simulink model "mcb_microchip_pmsm_parameter_est_SAME70"  (R2023b)
settings: Solver=FixedStepDiscrete  StartTime=0.0  StopTime=15  RelTol=1e-3  EnableMultiTasking=on
InitFcn:
  | mcb_microchip_pmsm_parameter_est_SAME70_data;
values from neighbouring files (symbols this model uses):
  Ts = T_pwm    (= 5e-05)    [mcb_microchip_pmsm_parameter_est_SAME70_data.m]
  Ts_motor = T_pwm/2    (= 2.5e-05)    [mcb_microchip_pmsm_parameter_est_SAME70_data.m]
undefined symbols (not defined in the file or in its folder): A24, AD10, AD7, ADC0, inverter, LQFP144, MaxPer, ms, ns, PA0, PA1, PA10, PA11, PA12, PA13, PA16, PA18, PA9, PB0, PD18, PD19, PD24, PD25, PD26, PI_params, Pin, pmsm, Resol, SAME70Q21B, target, Unsigned
libraries: simulink x18, MCHP_Blockset x13, mcbpmsmparamestlib x5, svdutilitieslib x4, mcbpositiondecoderlib x3, mcbplantlib x1, autolibpmsmexterior x1, mcbcontrolslib x1
(part 3 of 4)

== system mcb_microchip_pmsm_parameter_est_SAME70/Microcontroller/Heartbeat LED ==
  Codegen : Subsystem  VariantControl=(codegen)
  Sim : Subsystem  VariantControl=(sim)

== system mcb_microchip_pmsm_parameter_est_SAME70/Microcontroller/Input HW Drivers ==
  PhaseCurr_fb : Inport
  Position_fb : Inport  Port=2
  Codegen : Subsystem  VariantControl=(codegen)
  Sim : Subsystem  VariantControl=(sim)
  IabADC : Outport
  VdcADC : Outport  Port=2
  Vabc_ADC : Outport  Port=3
  eQEP : Outport  Port=4

== system mcb_microchip_pmsm_parameter_est_SAME70/Microcontroller/Input Scaling ==
  Mode : Inport
  Iab_ADC : Inport  Port=2
  Vdc_ADC : Inport  Port=3
  Vabc_ADC : Inport  Port=4
  Gain : Gain  Gain=inverter.VoltPerCount  OutDataTypeStr=dataType  RndMeth=Simplest
  Gain1 : Gain  Gain=inverter.VoltPerCount  OutDataTypeStr=dataType  RndMeth=Simplest
  Variant Subsystem : Subsystem  Variant=on
  Iab : Outport
  Vdc : Outport  Port=2
  Vabc : Outport  Port=3
  wires:
  Variant Subsystem/1(Iab) -> Iab/1
  Mode/1 -> Variant Subsystem/1(Mode)
  Iab_ADC/1 -> Variant Subsystem/2(Iab_ADC)
  Vdc_ADC/1 -> Gain/1
  Gain/1 -> Vdc/1
  Vabc_ADC/1 -> Gain1/1
  Gain1/1 -> Vabc/1

== system mcb_microchip_pmsm_parameter_est_SAME70/Microcontroller/Mode Control ==
  ClosedLoop : Subsystem  VariantControl=inverter.ADCOffsetCalibEnable == 0 && pmsm.QEPIndexPresent == true
  CurrentCalib : Subsystem  VariantControl=inverter.ADCOffsetCalibEnable == 1 && pmsm.QEPIndexPresent == true
  CurrentPosCalib : Subsystem  VariantControl=inverter.ADCOffsetCalibEnable == 1 && pmsm.QEPIndexPresent == false
  PosCalib : Subsystem  VariantControl=inverter.ADCOffsetCalibEnable == 0 && pmsm.QEPIndexPresent == false
  Mode : Outport

== system mcb_microchip_pmsm_parameter_est_SAME70/Microcontroller/Output PWM Drivers ==
  PWM_In : Inport
  InvEn : Inport  Port=2
  Codegen : Subsystem  VariantControl=(codegen)
  Sim : Subsystem  VariantControl=(sim)
  PWM : Outport

== system mcb_microchip_pmsm_parameter_est_SAME70/Microcontroller/Output Scaling ==
  Mode : Inport
  Vabc_Ref : Inport  Port=2
  InverterEn : Inport  Port=3
  Constant2 : Constant  OutDataTypeStr=dataType
  Current offset measurement : Constant  Value=[0 0 0]  OutDataTypeStr=dataType
  Mode1 : InportShadow
  Mode2 : InportShadow
  Position offset calibration : Constant  Value=[0.2 -0.1 -0.1]  OutDataTypeStr=dataType
  Switch : Switch  Threshold=1  SaturateOnIntegerOverflow=off  InputSameDT=off
  Switch1 : Switch  Threshold=2  SaturateOnIntegerOverflow=off  InputSameDT=off
  Switch2 : Switch  Threshold=2  SaturateOnIntegerOverflow=off  InputSameDT=off
  PWM : Outport
  InvEn : Outport  Port=2
  wires:
  Switch/1 -> PWM/1
  Switch1/1 -> InvEn/1
  Mode/1 -> Switch/2
  Current offset measurement/1 -> Switch/3
  Switch2/1 -> Switch/1
  Mode1/1 -> Switch2/2
  Vabc_Ref/1 -> Switch2/1
  Position offset calibration/1 -> Switch2/3
  InverterEn/1 -> Switch1/1
  Mode2/1 -> Switch1/2
  Constant2/1 -> Switch1/3

== system mcb_microchip_pmsm_parameter_est_SAME70/Microcontroller/SCI In Abstraction ==
  SCI_Data : Inport
  Mode : Inport  Port=2
  Variant Subsystem : Subsystem  Variant=on  VariantControlMode=sim codegen switching
  ConfigAndCommand : Outport
  DebugSel : Outport  Port=2
  wires:
  Variant Subsystem/1(ConfigAndCommand) -> ConfigAndCommand/1
  Variant Subsystem/2(DebugSel) -> DebugSel/1
  SCI_Data/1 -> Variant Subsystem/1(SCI_Data)
  Mode/1 -> Variant Subsystem/2(Mode)

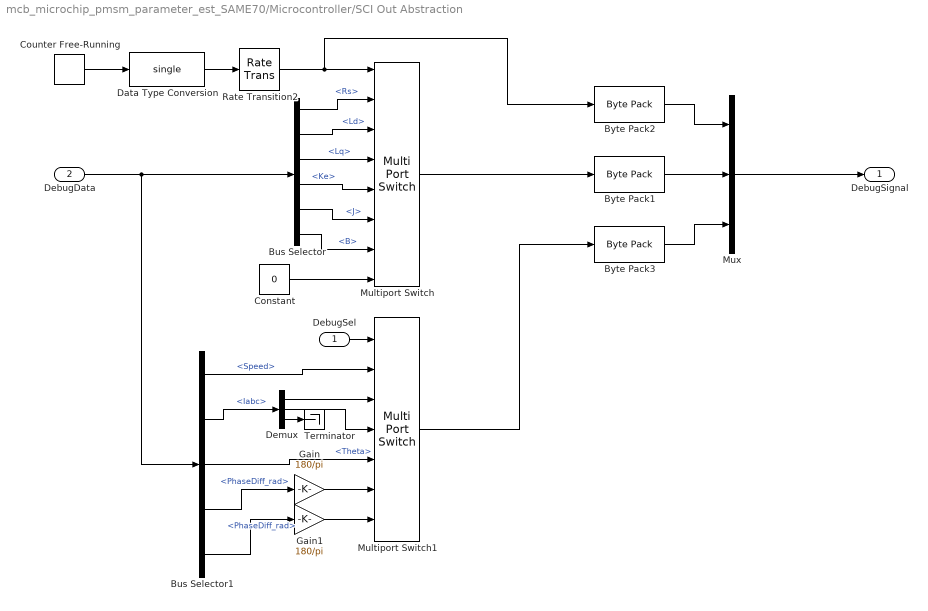
== system mcb_microchip_pmsm_parameter_est_SAME70/Microcontroller/SCI Out Abstraction ==
  DebugSel : Inport
  DebugData : Inport  Port=2
  Bus Selector : BusSelector  OutputSignals=MotorParams.Rs,MotorParams.Ld,MotorParams.Lq,MotorParams.Ke,MotorParams.J,MotorParams.B
  Bus Selector1 : BusSelector  OutputSignals=HWInputs.Speed,HWInputs.Iabc,HWInputs.Theta,LdLog.PhaseDiff_rad,LqLog.PhaseDiff_rad
  Byte Pack1 : svdutilitieslib/Byte Pack  maskPackedDataType=uint8  datatypes={'single'}  byteAlign=1  blockPlatform=tic2000
  Byte Pack2 : svdutilitieslib/Byte Pack  maskPackedDataType=uint8  datatypes={'single'}  byteAlign=1  blockPlatform=tic2000
  Byte Pack3 : svdutilitieslib/Byte Pack  maskPackedDataType=uint8  datatypes={'single'}  byteAlign=1  blockPlatform=tic2000
  Constant : Constant  Value=0  OutDataTypeStr=dataType
  Counter Free-Running : simulink/Sources/Counter Free-Running  NumBits=3  tsamp=0.5
  Data Type Conversion : DataTypeConversion  OutDataTypeStr=single  RndMeth=Simplest  SaturateOnIntegerOverflow=off
  Demux : Demux  Outputs=3
  Gain : Gain  Gain=180/pi
  Gain1 : Gain  Gain=180/pi
  Multiport Switch : MultiPortSwitch  Inputs=7  DiagnosticForDefault=None  SaturateOnIntegerOverflow=off  InputSameDT=off
  Multiport Switch1 : MultiPortSwitch  Inputs=6  DiagnosticForDefault=None  SaturateOnIntegerOverflow=off  InputSameDT=off
  Mux : Mux  Inputs=3
  Rate Transition2 : RateTransition  Deterministic=off  OutPortSampleTime=Ts
  Terminator : Terminator
  DebugSignal : Outport
  wires:
  Counter Free-Running/1 -> Data Type Conversion/1
  Data Type Conversion/1 -> Rate Transition2/1
  DebugData/1 -> Bus Selector1/1, Bus Selector/1
  Bus Selector/4 -> Multiport Switch/5  "<Ke>"
  Bus Selector/5 -> Multiport Switch/6  "<J>"
  Bus Selector/3 -> Multiport Switch/4  "<Lq>"
  Bus Selector/6 -> Multiport Switch/7  "<B>"
  Bus Selector/2 -> Multiport Switch/3  "<Ld>"
  Bus Selector/1 -> Multiport Switch/2  "<Rs>"
  Constant/1 -> Multiport Switch/8
  DebugSel/1 -> Multiport Switch1/1
  Multiport Switch/1 -> Byte Pack1/1
  Multiport Switch1/1 -> Byte Pack3/1
  Bus Selector1/1 -> Multiport Switch1/2  "<Speed>"
  Demux/1 -> Multiport Switch1/3
  Demux/2 -> Multiport Switch1/4
  Mux/1 -> DebugSignal/1
  Demux/3 -> Terminator/1
  Byte Pack2/1 -> Mux/1
  Byte Pack1/1 -> Mux/2
  Byte Pack3/1 -> Mux/3
  Rate Transition2/1 -> Byte Pack2/1, Multiport Switch/1
  Gain/1 -> Multiport Switch1/6
  Gain1/1 -> Multiport Switch1/7
  Bus Selector1/4 -> Gain/1  "<PhaseDiff_rad>"
  Bus Selector1/5 -> Gain1/1  "<PhaseDiff_rad>"
  Bus Selector1/2 -> Demux/1  "<Iabc>"
  Bus Selector1/3 -> Multiport Switch1/5  "<Theta>"

== system mcb_microchip_pmsm_parameter_est_SAME70/Microcontroller/SCI_Rx ==
  CodeGen : Subsystem
  Sim : Subsystem
  Variant Source : VariantSource  VariantControlMode=sim codegen switching
  Data : Outport
  wires:
  CodeGen/1(Data) -> Variant Source/1
  Variant Source/1 -> Data/1
  Sim/1(Data) -> Variant Source/2

== system mcb_microchip_pmsm_parameter_est_SAME70/Microcontroller/SCI_Tx ==
  SCI_Tx_Data : Inport
  Codegen : Subsystem  SystemSampleTime=0.03  VariantControl=(codegen)
  Sim : Subsystem  VariantControl=(sim)

== system mcb_microchip_pmsm_parameter_est_SAME70/Inverter and Motor/Inverter and Motor/Codegen ==
  Duty_Cycles : Inport
  Ground : Ground
  Terminator : Terminator
  PhaseCurr_fb : Outport
  Position_fb : Outport  Port=2
  wires:
  Duty_Cycles/1 -> Terminator/1
  Ground/1 -> PhaseCurr_fb/1, Position_fb/1

== system mcb_microchip_pmsm_parameter_est_SAME70/Inverter and Motor/Inverter and Motor/Sim ==
  Duty_Cycles : Inport
  Motor : Subsystem
  RT1 : RateTransition  Deterministic=off  OutPortSampleTime=Ts_simulink
  RT2 : RateTransition  Deterministic=off  OutPortSampleTime=Ts_simulink
  Rate Transition2 : RateTransition  Deterministic=off  OutPortSampleTime=Ts
  Rate Transition3 : RateTransition  Deterministic=off  OutPortSampleTime=Ts_inverter
  Rate Transition4 : RateTransition  Deterministic=off  OutPortSampleTime=Ts
  Sensor Measurements : Subsystem
  PhaseCurr_fb : Outport
  Position_fb : Outport  Port=2
  wires:
  RT1/1 -> Sensor Measurements/2(PhaseCurr)
  Duty_Cycles/1 -> Rate Transition3/1
  Sensor Measurements/2(Position_fb) -> Rate Transition4/1
  Sensor Measurements/1(PhaseCurr_fb) -> Rate Transition2/1
  Rate Transition2/1 -> PhaseCurr_fb/1
  Rate Transition4/1 -> Position_fb/1
  RT2/1 -> Sensor Measurements/1(Info)
  Rate Transition3/1 -> Motor/1(Duty_Cycles)
  Motor/1(ThetaMech) -> RT2/1
  Motor/2(Iabc) -> RT1/1

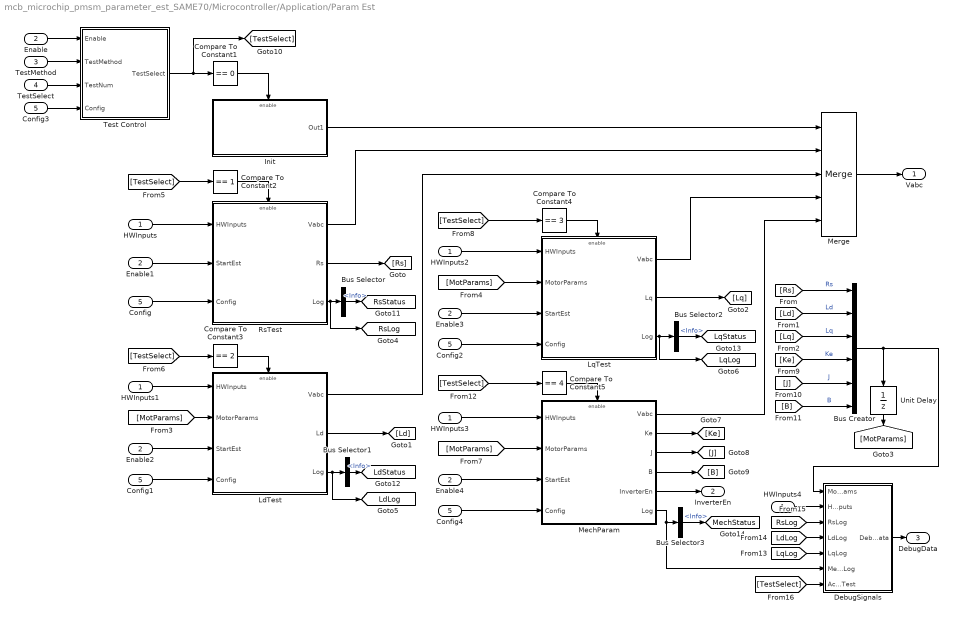
== system mcb_microchip_pmsm_parameter_est_SAME70/Microcontroller/Application/Param Est ==
  HWInputs : Inport
  Enable : Inport  Port=2
  TestMethod : Inport  Port=3
  TestSelect : Inport  Port=4
  Config : Inport  Port=5
  Bus Creator : BusCreator  Inputs=6
  Bus Selector{,1..3} (4 alike) : BusSelector  OutputSignals=Info
  Compare To Constant1 : simulink/Logic and Bit Operations/Compare To Constant  relop===  const=0  OutDataTypeStr=boolean
  Compare To Constant2 : simulink/Logic and Bit Operations/Compare To Constant  relop===  const=1  OutDataTypeStr=boolean
  Compare To Constant3 : simulink/Logic and Bit Operations/Compare To Constant  relop===  const=2  OutDataTypeStr=boolean
  Compare To Constant4 : simulink/Logic and Bit Operations/Compare To Constant  relop===  const=3  OutDataTypeStr=boolean
  Compare To Constant5 : simulink/Logic and Bit Operations/Compare To Constant  relop===  const=4  OutDataTypeStr=boolean
  Config{1..4} (4 alike) : InportShadow  Port=5
  DebugSignals : Subsystem
  Enable{1..4} (4 alike) : InportShadow  Port=2
  HWInputs{1..4} (4 alike) : InportShadow
  Init : Subsystem
  LdTest : Subsystem
  LqTest : Subsystem
  MechParam : Subsystem
  Merge : Merge  Inputs=5
  RsTest : Subsystem
  Test Control : Subsystem
  Unit Delay : UnitDelay  SampleTime=-1  HasFrameUpgradeWarning=on
  Vabc : Outport
  InverterEn : Outport  Port=2
  DebugData : Outport  Port=3
  tag scope: LdLog=global, LdStatus=global, LqLog=global, LqStatus=global, MechStatus=global, RsLog=global, RsStatus=global
  wires:
  Config/1 -> RsTest/3(Config)
  Config1/1 -> LdTest/4(Config)
  Config2/1 -> LqTest/4(Config)
  HWInputs/1 -> RsTest/1(HWInputs)
  HWInputs1/1 -> LdTest/1(HWInputs)
  HWInputs2/1 -> LqTest/1(HWInputs)
  Bus Creator/1 -> Unit Delay/1, DebugSignals/1(MotorParams)
  RsTest/2(Rs) -> [Rs]
  LdTest/3(Log) -> [LdLog], Bus Selector1/1
  LdTest/2(Ld) -> [Ld]
  LqTest/2(Lq) -> [Lq]
  LqTest/3(Log) -> [LqLog], Bus Selector2/1
  [Rs] -> Bus Creator/1  "Rs"
  [Ld] -> Bus Creator/2  "Ld"
  [Lq] -> Bus Creator/3  "Lq"
  Unit Delay/1 -> [MotParams]
  [MotParams] -> LdTest/2(MotorParams)
  [MotParams] -> LqTest/2(MotorParams)
  Test Control/1(TestSelect) -> [TestSelect], Compare To Constant1/1
  Compare To Constant1/1 -> Init/Enable
  Compare To Constant2/1 -> RsTest/Enable
  Compare To Constant3/1 -> LdTest/Enable
  Compare To Constant4/1 -> LqTest/Enable
  Bus Selector1/1 -> [LdStatus]  "<Info>"
  Bus Selector2/1 -> [LqStatus]  "<Info>"
  Compare To Constant5/1 -> MechParam/Enable
  HWInputs3/1 -> MechParam/1(HWInputs)
  Config4/1 -> MechParam/4(Config)
  [MotParams] -> MechParam/2(MotorParams)
  MechParam/6(Log) -> DebugSignals/6(MechLog), Bus Selector3/1
  MechParam/2(Ke) -> [Ke]
  [Ke] -> Bus Creator/4  "Ke"
  Merge/1 -> Vabc/1
  Init/1(Out1) -> Merge/1
  RsTest/1(Vabc) -> Merge/2
  LdTest/1(Vabc) -> Merge/3
  LqTest/1(Vabc) -> Merge/4
  MechParam/1(Vabc) -> Merge/5
  MechParam/3(J) -> [J]
  MechParam/4(B) -> [B]
  [J] -> Bus Creator/5  "J"
  [B] -> Bus Creator/6  "B"
  MechParam/5(InverterEn) -> InverterEn/1
  Enable/1 -> Test Control/1(Enable)
  TestSelect/1 -> Test Control/3(TestNum)
  TestMethod/1 -> Test Control/2(TestMethod)
  [TestSelect] -> Compare To Constant2/1
  [TestSelect] -> Compare To Constant3/1
  [TestSelect] -> Compare To Constant4/1
  [TestSelect] -> Compare To Constant5/1
  Enable1/1 -> RsTest/2(StartEst)
  Enable2/1 -> LdTest/3(StartEst)
  Enable3/1 -> LqTest/3(StartEst)
  Enable4/1 -> MechParam/3(StartEst)
  Bus Selector/1 -> [RsStatus]  "<Info>"
  Bus Selector3/1 -> [MechStatus]  "<Info>"
  HWInputs4/1 -> DebugSignals/2(HWInputs)
  RsTest/3(Log) -> [RsLog], Bus Selector/1
  [LqLog] -> DebugSignals/5(LqLog)
  [LdLog] -> DebugSignals/4(LdLog)
  [RsLog] -> DebugSignals/3(RsLog)
  DebugSignals/1(DebugData) -> DebugData/1
  Config3/1 -> Test Control/4(Config)
  [TestSelect] -> DebugSignals/7(ActiveTest)

== system mcb_microchip_pmsm_parameter_est_SAME70/Microcontroller/Application Abstraction/Variant Subsystem ==
  eQEPCnt : Inport
  eQEPIndex : Inport  Port=2
  Mode : Inport  Port=3
  Index Absent : Subsystem  VariantControl=pmsm.QEPIndexPresent == false
  Index Present : Subsystem  VariantControl=pmsm.QEPIndexPresent == true
  Theta : Outport
  Speed : Outport  Port=2
  EnClosedLoop : Outport  Port=3

== system mcb_microchip_pmsm_parameter_est_SAME70/Microcontroller/Heartbeat LED/Codegen ==
  DBG LED 1 : MCHP_Blockset/Digital IO/Digital Output Write  PORT=Dynamic Options  PORT_TXT="C   [ 0 : 31 ]"  PIN=23  PACK=off  SIMULTANEOUS=off  ORDERING=None  SampleTime=-1  MCHP_PORT={Digital Out}{DOU}1:1:C23;  MCHP_MASTERLINK=mcb_microchip_pmsm_parameter_est_SAME70_23b_lib/Microcontroller/Configurations/Microchip Master
      settings: SourceProductName=MPLAB Device Blocks for Simulink
  Delay 10Hz : Delay  DelayLength=1  InitialCondition=0  SampleTime=0.25
  Logical Operator : Logic  Operator=NOT  AllPortsSameDT=off  OutDataTypeStr=boolean
  wires:
  Delay 10Hz/1 -> Logical Operator/1
  Logical Operator/1 -> DBG LED 1/1, Delay 10Hz/1

== system mcb_microchip_pmsm_parameter_est_SAME70/Microcontroller/Heartbeat LED/Sim ==

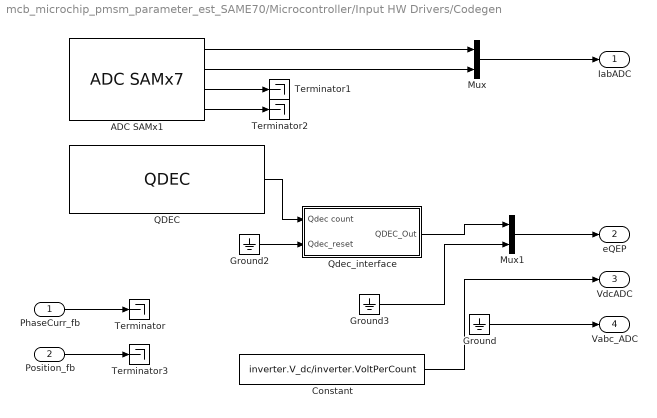
== system mcb_microchip_pmsm_parameter_est_SAME70/Microcontroller/Input HW Drivers/Codegen ==
  PhaseCurr_fb : Inport
  Position_fb : Inport  Port=2
  ADC SAMx1 : MCHP_Blockset/Analog IO/ADC SAMx7  Priority=-2000  AFECx=AFE Controller 0  SIGNMODE_SingleEnded=Unsigned (uint16)  SIGNMODE_Differential=Unsigned (uint16)  AFEC0_seq0=Dynamic Options  AFEC0_seq0_TXT="AD0 / PD30   &   AD6 / PA17"  AFEC1_seq0=Dynamic Options  AFEC1_seq0_TXT=Not used  AFEC0_seq1=Dynamic Options  AFEC0_seq1_TXT=AD7 / PA18  AFEC1_seq1=Dynamic Options  AFEC1_seq1_TXT=Not used  AFEC0_seq2=Dynamic Options  AFEC0_seq2_TXT=AD10 / PB0  AFEC1_seq2=Dynamic Options  AFEC1_seq2_TXT=Not used  AFEC0_seq3=Dynamic Options  AFEC0_seq3_TXT=Not used  AFEC1_seq3=Dynamic Options  AFEC1_seq3_TXT=Not used  AFEC0_seq4=Dynamic Options  AFEC0_seq4_TXT=Not used  AFEC1_seq4=Dynamic Options  AFEC1_seq4_TXT=Not used  AFEC0_seq5=Dynamic Options  AFEC0_seq5_TXT=Not used  AFEC1_seq5=Dynamic Options  AFEC1_seq5_TXT=Not used  AFEC0_seq6=Dynamic Options  AFEC0_seq6_TXT=Not used  AFEC1_seq6=Dynamic Options  AFEC1_seq6_TXT=Not used  AFEC0_seq7=Dynamic Options  AFEC0_seq7_TXT=Not used  AFEC1_seq7=Dynamic Options  AFEC1_seq7_TXT=Not used  AFEC0_seq8=Dynamic Options  AFEC0_seq8_TXT=Not used  AFEC1_seq8=Dynamic Options  AFEC1_seq8_TXT=Not used  AFEC0_seq9=Dynamic Options  AFEC0_seq9_TXT=Not used  AFEC1_seq9=Dynamic Options  AFEC1_seq9_TXT=Not used  AFEC0_seq10=Dynamic Options  AFEC0_seq10_TXT=Not used  AFEC1_seq10=Dynamic Options  AFEC1_seq10_TXT=Not used  AFEC0_seq11=Dynamic Options  AFEC0_seq11_TXT=Not used  AFEC1_seq11=Dynamic Options  AFEC1_seq11_TXT=Not used  SampleTime=Ts  S_INPUT=[-1]  S_INPUT_Size=[3]  S_OUTPUT=[]  S_OUTPUT_Size=[]  S_ListCustomDatatype=S.S_ListCustomDatatype={};  MCHP_AFECC_CLOCK_REQUEST=''  MCHP_AFECC_CLOCK_RESULT=''  MCHP_USER_INTERRUPTS=0  MCHP_PORT={AD0 AFEC0}{AD0}15:2:P126;{AD6 AFEC0}{AD6}15:2:P17;{AD7 AFEC0}{AD7}15:2:P18;{AD10 AFEC0}{AD10}15:2:P32;  MCHP_MASTERLINK=mcb_microchip_pmsm_parameter_est_SAME70_23b_lib/Microcontroller/Configurations/Microchip Master  Rin=< 200 Ohm  RES=12-bit Standard  AFEC0_Synchronisation=Triggered by user defined source  AFEC0_Trig=PWM0 event line 0  AFEC0_TrigTimeStep=on  AFEC1_Synchronisation=Triggered by user defined source  AFEC1_Trig=PWM1 event line 0  AFEC1_TrigTimeStep=off  ADC_TrigInfo=0  AFEC0_seq0_GAIN=1  AFEC1_seq0_GAIN=1  AFEC0_seq1_GAIN=1  AFEC1_seq1_GAIN=1  AFEC0_seq2_GAIN=1  AFEC1_seq2_GAIN=1  AFEC0_seq3_GAIN=1  AFEC1_seq3_GAIN=1  AFEC0_seq4_GAIN=1  AFEC1_seq4_GAIN=1  AFEC0_seq5_GAIN=1  AFEC1_seq5_GAIN=1  AFEC0_seq6_GAIN=1  AFEC1_seq6_GAIN=1  AFEC0_seq7_GAIN=1  AFEC1_seq7_GAIN=1  AFEC0_seq8_GAIN=1  AFEC1_seq8_GAIN=1  AFEC0_seq9_GAIN=1  AFEC1_seq9_GAIN=1  AFEC0_seq10_GAIN=1  AFEC1_seq10_GAIN=1  AFEC0_seq11_GAIN=1  AFEC1_seq11_GAIN=1  AFEC0_seq0_OFFSET=0  AFEC1_seq0_OFFSET=0  AFEC0_seq1_OFFSET=0  AFEC1_seq1_OFFSET=0  AFEC0_seq2_OFFSET=0  AFEC1_seq2_OFFSET=0  AFEC0_seq3_OFFSET=0  AFEC1_seq3_OFFSET=0  AFEC0_seq4_OFFSET=0  AFEC1_seq4_OFFSET=0  AFEC0_seq5_OFFSET=0  AFEC1_seq5_OFFSET=0  AFEC0_seq6_OFFSET=0  AFEC1_seq6_OFFSET=0  AFEC0_seq7_OFFSET=0  AFEC1_seq7_OFFSET=0  AFEC0_seq8_OFFSET=0  AFEC1_seq8_OFFSET=0  AFEC0_seq9_OFFSET=0  AFEC1_seq9_OFFSET=0  AFEC0_seq10_OFFSET=0  AFEC1_seq10_OFFSET=0  AFEC0_seq11_OFFSET=0  AFEC1_seq11_OFFSET=0
      settings: SourceProductName=MPLAB Device Blocks for Simulink
  Constant : Constant  Value=inverter.V_dc/inverter.VoltPerCount  OutDataTypeStr=uint16
  Ground : Ground
  Ground2 : Ground
  Ground3 : Ground
  Mux : Mux  Inputs=2
  Mux1 : Mux  Inputs=2
  QDEC : MCHP_Blockset/QEI/QDEC  QDEC_REF=Dynamic Options  QDEC_REF_TXT=TC0  PHA_PIN=Dynamic Options  PHA_PIN_TXT=PA0 / Pin[102]  PHB_PIN=Dynamic Options  PHB_PIN_TXT=PA1 / Pin[99]  IDX_PIN=Dynamic Options  IDX_PIN_TXT=PA16 / Pin[45]  INVERT_PHA=off  INVERT_PHB=off  INVERT_IDX=off  SWAP_PHA_PHB=off  SampleTime=Ts  MCHP_PORT={TC0}{TIOA0}3:0:P0;{TC0}{TIOB0}3:0:P1;{TC0}{TIOB1}3:0:P16;  MCHP_MASTERLINK=mcb_microchip_pmsm_parameter_est_SAME70_23b_lib/Microcontroller/Configurations/Microchip Master  MCHP_TIMER_REQUEST={Quadrature Decoder (Phase Counter)}{QDEC0}20:4:4:0:[1]:65535;{Quadrature Decoder (IDX Counter)}{QDEC0}20:4:4:0:[2]:65535;{Quadrature Decoder (Speed Measurement Time Base)}{QDEC0}20:4:4:0:[3]:65535;  MCHP_TIMER_RESULT=[1 65535]  QDEC_MODE=Position  POSITION_OUTPUT=is a 16 bits unsigned block output  INDEX_OUTPUT=is not a block output  RESET_INPUT=off  POSITION_RESET_MODE=never reset position  RESET_EDGE=rising edge  POSITION_RESET_VALUE=65535  SPEED_TIME_BASE=Dynamic Options  SPEED_TIME_BASE_TXT=Resol: 53.33(ns) - MaxPer: 3.5(ms)  SPEED_OUTPUT=is a 16 bits unsigned block output  DIR_OUTPUT=is not a block output  DIRCHG_OUTPUT=is not a block output  AUTO_CORRECTION=off  MAX_PERIOD_FILTER=Dynamic Options  MAX_PERIOD_FILTER_TXT=420(ns)  MAXCMP=disabled  MPE_OUTPUT=is not a block output  QERR_OUTPUT=is not a block output
      settings: SourceProductName=MPLAB Device Blocks for Simulink
  Qdec_interface : Subsystem  mask{EnCountPerRev=pmsm.QEPSlits*4}
      mask prompts: EnCountPerRev "Encoder counts per rev"
  Terminator{,1..3} (4 alike) : Terminator
  IabADC : Outport
  eQEP : Outport  Port=2
  VdcADC : Outport  Port=3
  Vabc_ADC : Outport  Port=4
  wires:
  ADC SAMx1/4 -> Terminator2/1
  ADC SAMx1/3 -> Terminator1/1
  Ground2/1 -> Qdec_interface/2(Qdec_reset)
  QDEC/1 -> Qdec_interface/1(Qdec count)
  PhaseCurr_fb/1 -> Terminator/1
  Position_fb/1 -> Terminator3/1
  Ground/1 -> Vabc_ADC/1
  Constant/1 -> VdcADC/1
  ADC SAMx1/1 -> Mux/1
  ADC SAMx1/2 -> Mux/2
  Mux/1 -> IabADC/1
  Qdec_interface/1(QDEC_Out) -> Mux1/1
  Mux1/1 -> eQEP/1
  Ground3/1 -> Mux1/2

== system mcb_microchip_pmsm_parameter_est_SAME70/Microcontroller/Input HW Drivers/Sim ==
  PhaseCurr_fb : Inport
  Position_fb : Inport  Port=2
  Constant : Constant  Value=inverter.V_dc/inverter.VoltPerCount  OutDataTypeStr=uint16
  Ground : Ground
  IabADC : Outport
  eQEP : Outport  Port=2
  VdcADC : Outport  Port=3
  Vabc_ADC : Outport  Port=4
  wires:
  PhaseCurr_fb/1 -> IabADC/1
  Position_fb/1 -> eQEP/1
  Ground/1 -> Vabc_ADC/1
  Constant/1 -> VdcADC/1

== system mcb_microchip_pmsm_parameter_est_SAME70/Microcontroller/Input Scaling/Variant Subsystem ==
  Mode : Inport
  Iab_ADC : Inport  Port=2
  Automatic offset calibration : Subsystem  VariantControl=inverter.ADCOffsetCalibEnable == 1
  Offser via parameter : Subsystem  VariantControl=inverter.ADCOffsetCalibEnable == 0
  Iab : Outport

== system mcb_microchip_pmsm_parameter_est_SAME70/Microcontroller/Mode Control/ClosedLoop ==
  Constant : Constant  Value=2  OutDataTypeStr=single  SampleTime=0.1
  Mode : Outport
  wires:
  Constant/1 -> Mode/1

== system mcb_microchip_pmsm_parameter_est_SAME70/Microcontroller/Mode Control/CurrentCalib ==
  Step : Step  After=2  OutDataTypeStr=single  SampleTime=0.1
  Mode : Outport
  wires:
  Step/1 -> Mode/1

== system mcb_microchip_pmsm_parameter_est_SAME70/Microcontroller/Mode Control/CurrentPosCalib ==
  Add : Sum
  Step : Step  OutDataTypeStr=single  SampleTime=0.1
  Step1 : Step  Time=2  OutDataTypeStr=single  SampleTime=0.1
  Mode : Outport
  wires:
  Step/1 -> Add/1
  Step1/1 -> Add/2
  Add/1 -> Mode/1

== system mcb_microchip_pmsm_parameter_est_SAME70/Microcontroller/Mode Control/PosCalib ==
  Step : Step  Before=1  After=2  OutDataTypeStr=single  SampleTime=0.1
  Mode : Outport
  wires:
  Step/1 -> Mode/1

== system mcb_microchip_pmsm_parameter_est_SAME70/Microcontroller/Output PWM Drivers/Codegen ==
  PWM_In : Inport
  InvEn : Inport  Port=2
  Constant : Constant  Value=0xF000F  OutDataTypeStr=uint32  SampleTime=-1
  Constant1 : Constant  Value=0  OutDataTypeStr=uint32  SampleTime=-1
  Constant2 : Constant  Value=0  OutDataTypeStr=uint32  SampleTime=-1
  Data Type Conversion : DataTypeConversion  OutDataTypeStr=single  SaturateOnIntegerOverflow=off  RndMeth=Floor
  Ground : Ground
  InvEn1 : InportShadow  Port=2
  Mux3 : Mux  Inputs=3
  PWM SAM7x : MCHP_Blockset/PWM IO/PWM SAM7x  Priority=-2000  PWMx=PWM Controller 0  MaxPeriod_s=Ts  PWM0_pinH0=Dynamic Options  PWM0_pinH0_TXT=PA11 / Pin[64]  PWM0_pinL0=Dynamic Options  PWM0_pinL0_TXT=PD24 / Pin[55]  PWM0_pinH1=Dynamic Options  PWM0_pinH1_TXT=PA12 / Pin[68]  PWM0_pinL1=Dynamic Options  PWM0_pinL1_TXT=PD25 / Pin[52]  PWM0_pinH2=Dynamic Options  PWM0_pinH2_TXT=PA13 / Pin[42]  PWM0_pinL2=Dynamic Options  PWM0_pinL2_TXT=PD26 / Pin[53]  PWM0_pinH3=Dynamic Options  PWM0_pinH3_TXT=Not Used  PWM0_pinL3=Dynamic Options  PWM0_pinL3_TXT=Not Used  PWM1_pinH0=Dynamic Options  PWM1_pinH0_TXT=Not Used  PWM1_pinL0=Dynamic Options  PWM1_pinL0_TXT=Not Used  PWM1_pinH1=Dynamic Options  PWM1_pinH1_TXT=Not Used  PWM1_pinL1=Dynamic Options  PWM1_pinL1_TXT=Not Used  PWM1_pinH2=Dynamic Options  PWM1_pinH2_TXT=Not Used  PWM1_pinL2=Dynamic Options  PWM1_pinL2_TXT=Not Used  PWM1_pinH3=Dynamic Options  PWM1_pinH3_TXT=Not Used  PWM1_pinL3=Dynamic Options  PWM1_pinL3_TXT=Not Used  PWM_Centered=on  PWM_SyncWithPWM0=on  PushPull_Mode=off  SampleTime=Ts  S_INPUT=[-1]  S_INPUT_Size=[3]  S_OUTPUT=[]  S_OUTPUT_Size=[]  S_ListCustomDatatype=S.S_ListCustomDatatype={};  evalin_ws=PWM0max0=MCHP_Fun.Hex2num('40AD4C0000000000');PWM1max0=MCHP_Fun.Hex2num('40AD4C0000000000');PWM2max0=MCHP_Fun.Hex2num('40AD4C0000000000');  MCHP_PWMC_CLOCK_REQUEST=''  MCHP_PWMC_CLOCK_RESULT=''  MCHP_USER_INTERRUPTS=0  MCHP_PORT={PWM0H0 }{PWMH0}4:1:P11;{PWM0L0 }{PWML0}4:1:P120;{PWM0H1 }{PWMH1}4:1:P12;{PWM0L1 }{PWML1}4:1:P121;{PWM0H2 }{PWMH2}4:1:P13;{PWM0L2 }{PWML2}4:1:P122;  MCHP_MASTERLINK=mcb_microchip_pmsm_parameter_est_SAME70_23b_lib/Microcontroller/Configurations/Microchip Master  invert_PWMH0=off  invert_PWML0=off  invert_PWMH1=off  invert_PWML1=off  invert_PWMH2=off  invert_PWML2=off  invert_PWMH3=off  invert_PWML3=off  InitPeriod_s=Ts  InitDutyCycle_s=0  InitDeadTimeH_s=1e-6  InitDeadTimeL_s=1e-6  InitEventLine0_ComparatorValue_s=1e-7  InitEventLine1_ComparatorValue_s=[]  BlockInput_VectorScalar=Vectors (grouped by function)  BlockInput_Period=Not a block input  BlockInput_DutyCycle=a Floating Point input within range [-1 1]  BlockInput_DeadTime=Not a block input  BlockInput_OutputOverride=Not a block input  Fault_FPV0=Not forced  Fault_FPV1=Not forced  Fault_FPV2=Not forced  Fault_FPV3=Not forced  Fault_Input0=does nothing  Fault_Input0_FFIL=off  Fault_Input1=does nothing  Fault_Input1_FFIL=off  Fault_Input2=does nothing  Fault_Input2_FFIL=on  Fault_Input3=does nothing  Fault_Input3_FFIL=off  Fault_Input4=does nothing  Fault_Input4_FFIL=on  Fault_Input5=does nothing  Fault_Input5_FFIL=on  Fault_Input6=does nothing  Fault_Input6_FFIL=on  Fault_Input7=does nothing  Fault_Input7_FFIL=on
      settings: SourceProductName=MPLAB Device Blocks for Simulink
  PWM SAM7x Output Override : MCHP_Blockset/PWM IO/PWM SAM7x  Output Override  Priority=-2000  PWMx=PWM Controller 0  SampleTime=Ts  S_INPUT=[-1]  S_INPUT_Size=[3]  S_OUTPUT=[]  S_OUTPUT_Size=[]  S_ListCustomDatatype=S.S_ListCustomDatatype={};  MCHP_MASTERLINK=mcb_microchip_pmsm_parameter_est_SAME70_23b_lib/Microcontroller/Configurations/Microchip Master  Init_PWM_OS=0x0000  Init_PWM_OOV=0x0000  Input_PWM_OS=on  Input_PWM_OS_off=off  Input_PWM_OSS=off  Input_PWM_OSS_off=off  Input_PWM_OSSUPD=off  Input_PWM_OSSUPD_off=off  Input_PWM_OSC=off  Input_PWM_OSC_off=off  Input_PWM_OSCUPD=off  Input_PWM_OSCUPD_off=off  Input_PWM_OOV=on
      settings: SourceProductName=MPLAB Device Blocks for Simulink
  Switch1 : Switch  Threshold=0.5  RndMeth=Simplest  SaturateOnIntegerOverflow=off  InputSameDT=off
  Switch4 : Switch  Threshold=0.5  RndMeth=Simplest  SaturateOnIntegerOverflow=off  InputSameDT=off
  stop : Constant  Value=0  OutDataTypeStr=dataType
  PWM : Outport
  wires:
  Mux3/1 -> Switch4/3
  Switch4/1 -> Data Type Conversion/1
  Data Type Conversion/1 -> PWM SAM7x/1
  stop/1 -> Mux3/3, Mux3/2, Mux3/1
  Ground/1 -> PWM/1
  InvEn/1 -> Switch4/2
  PWM_In/1 -> Switch4/1
  Constant1/1 -> Switch1/1
  Switch1/1 -> PWM SAM7x Output Override/1
  Constant2/1 -> PWM SAM7x Output Override/2
  Constant/1 -> Switch1/3
  InvEn1/1 -> Switch1/2

== system mcb_microchip_pmsm_parameter_est_SAME70/Microcontroller/Output PWM Drivers/Sim ==
  PWM_In : Inport
  InvEn : Inport  Port=2
  Mux2 : Mux  Inputs=3
  Subsystem : Subsystem
  Switch1 : Switch  Threshold=0.5  RndMeth=Simplest  SaturateOnIntegerOverflow=off  InputSameDT=off
  stop : Constant  Value=0  OutDataTypeStr=Inherit: Inherit via back propagation
  PWM : Outport
  wires:
  Mux2/1 -> Switch1/3
  stop/1 -> Mux2/1, Mux2/3, Mux2/2
  Subsystem/1(PWM_Duty_Cycles) -> Switch1/1
  Switch1/1 -> PWM/1
  InvEn/1 -> Switch1/2
  PWM_In/1 -> Subsystem/1(PWM_In)

== system mcb_microchip_pmsm_parameter_est_SAME70/Microcontroller/SCI In Abstraction/Variant Subsystem ==
  SCI_Data : Inport
  Mode : Inport  Port=2
  Codegen : Subsystem  VariantControl=(codegen)
  Sim : Subsystem  VariantControl=(sim)
  ConfigAndCommand : Outport
  DebugSel : Outport  Port=2

== system mcb_microchip_pmsm_parameter_est_SAME70/Microcontroller/SCI_Rx/CodeGen ==
  Data Type Conversion : DataTypeConversion  OutDataTypeStr=uint16  SaturateOnIntegerOverflow=off  RndMeth=Floor
  Subsystem : Subsystem
  Subsystem1 : Subsystem
  UART Rx : MCHP_Blockset/BUS UART/UART Rx  UART_REF=UART 0  Flag_Out=on  Rx_Size_popup=User defined  Rx_Size=1  S_Rx_Size=1  Split=Read all received char  SplitChar=10  OutputDefault_popup=do nothing (end of output vector will be undefined)  OutputDefault=-2  ORDERING=None  SampleTime=0.001  MCHP_MASTERLINK=mcb_microchip_pmsm_parameter_est_SAME70_23b_lib/Microcontroller/Configurations/Microchip Master  MCHP_COMPILED_INFO="CompiledSampleTime= [0.0010000000000000000208   0 ];CompiledInportDataTypes=[    ];CompiledInportDataWidth=[];"
      settings: SourceProductName=MPLAB Device Blocks for Simulink
  Data : Outport
  wires:
  UART Rx/1 -> Data Type Conversion/1
  UART Rx/2 -> Subsystem1/1(In1)
  Subsystem1/2(Data out) -> Subsystem/1(In1)
  Subsystem1/1(NewData) -> Subsystem/Enable
  Data Type Conversion/1 -> Subsystem1/Enable
  Subsystem/1(Data) -> Data/1

== system mcb_microchip_pmsm_parameter_est_SAME70/Microcontroller/SCI_Rx/Sim ==
  Constant : Constant  OutDataTypeStr=single
  Data : Outport
  wires:
  Constant/1 -> Data/1

== system mcb_microchip_pmsm_parameter_est_SAME70/Microcontroller/SCI_Tx/Codegen ==
  SCI_Tx_Data : Inport
  Counter Limited : simulink/Sources/Counter Limited  uplimit=target.SerialFrameSize-1  tsamp=-1
  Data : Subsystem  TreatAsAtomicUnit=on
  End : Subsystem  TreatAsAtomicUnit=on
  If : If  IfExpression=u1 == 0  ElseIfExpressions=u1 == single(target.SerialFrameSize-1)
  Start : Subsystem  TreatAsAtomicUnit=on
  wires:
  If/1 -> Start/Action
  SCI_Tx_Data/1 -> End/1(Data), Data/1(Data), Start/1(Data)
  If/2 -> End/Action
  Counter Limited/1 -> If/1
  If/3 -> Data/Action

== system mcb_microchip_pmsm_parameter_est_SAME70/Microcontroller/SCI_Tx/Sim ==
  SCI_Tx_Data : Inport
  Terminator : Terminator
  wires:
  SCI_Tx_Data/1 -> Terminator/1

== system mcb_microchip_pmsm_parameter_est_SAME70/Inverter and Motor/Inverter and Motor/Sim/Motor ==
  Duty_Cycles : Inport
  Bus Selector : BusSelector  OutputSignals=MtrPos
  Inverter : Subsystem
  Load_Profile (Torque) : Constant  Value=0  OutDataTypeStr=single
  Rate Transition1 : RateTransition  Deterministic=off  OutPortSampleTime=Ts_motor
  Surface Mount PMSM : autolibpmsmexterior/Surface Mount PMSM  port_config=Torque  sim_type=Discrete  Ts=Ts_motor  FilePath=surfacepmsm_motordata.m  P=pmsm.p  Rs=pmsm.Rs + inverter.R_board  Ldq_=pmsm.Ld  KConstText=Permanent flux linkage constant (lambda_pm):  lambda_pm=pmsm.FluxPM  Ke=159.9771  Kt=1.323  mechanical=[pmsm.J, pmsm.B, 0]  idq0=[0 0]  theta_init=0  omega_init=0  KConst=pmsm.FluxPM  lambda_pm_calc=pmsm.FluxPM  RefBlkName='autolibpmsmexterior/Surface Mount PMSM'  aMode=5  Ldq="[0.00078136  0.00078136]"
  Terminator : Terminator
  ThetaMech : Outport
  Iabc : Outport  Port=2
  wires:
  Bus Selector/1 -> ThetaMech/1  "<MtrPos>"
  Surface Mount PMSM/2 -> Iabc/1  "Iabc"
  Load_Profile (Torque)/1 -> Rate Transition1/1
  Duty_Cycles/1 -> Inverter/1(Duty_abc)
  Surface Mount PMSM/3 -> Terminator/1
  Surface Mount PMSM/1 -> Bus Selector/1
  Inverter/1(Vabc) -> Surface Mount PMSM/2
  Rate Transition1/1 -> Surface Mount PMSM/1

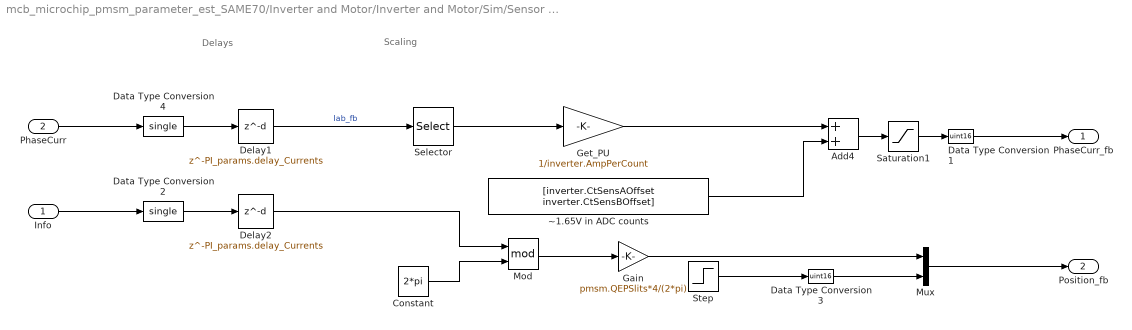
== system mcb_microchip_pmsm_parameter_est_SAME70/Inverter and Motor/Inverter and Motor/Sim/Sensor Measurements ==
  note: Scaling
  note: Delays
  Info : Inport
  PhaseCurr : Inport  Port=2
  Add4 : Sum  OutDataTypeStr=uint16
  Constant : Constant  Value=2*pi  OutDataTypeStr=Inherit: Inherit via back propagation  SampleTime=-1
  Data Type Conversion1 : DataTypeConversion  OutDataTypeStr=uint16  SaturateOnIntegerOverflow=off  RndMeth=Floor
  Data Type Conversion2 : DataTypeConversion  OutDataTypeStr=single  RndMeth=Simplest  SaturateOnIntegerOverflow=off
  Data Type Conversion3 : DataTypeConversion  OutDataTypeStr=uint16  SaturateOnIntegerOverflow=off  RndMeth=Floor
  Data Type Conversion4 : DataTypeConversion  OutDataTypeStr=single  RndMeth=Simplest  SaturateOnIntegerOverflow=off
  Delay1 : Delay  DelayLength=PI_params.delay_Currents
  Delay2 : Delay  DelayLength=PI_params.delay_Currents
  Gain : Gain  Gain=pmsm.QEPSlits*4/(2*pi)  OutDataTypeStr=uint16  RndMeth=Simplest
  Get_PU : Gain  Gain=1/inverter.AmpPerCount  OutDataTypeStr=int16  RndMeth=Simplest
  Mod : Math  Operator=mod
  Mux : Mux  Inputs=2
  Saturation1 : Saturate  UpperLimit=4095  LowerLimit=0
  Selector : Selector  InputPortWidth=3  IndexOptions=Index vector (dialog)  Indices=[1 2]  OutputSizes=1
  Step : Step  Time=0.01  OutDataTypeStr=single  SampleTime=0
  ~1.65V in ADC counts : Constant  Value=[inverter.CtSensAOffset inverter.CtSensBOffset]  OutDataTypeStr=uint16  SampleTime=-1
  PhaseCurr_fb : Outport
  Position_fb : Outport  Port=2
  wires:
  Saturation1/1 -> Data Type Conversion1/1
  Add4/1 -> Saturation1/1
  ~1.65V in ADC counts/1 -> Add4/2
  Delay1/1 -> Selector/1  "Iab_fb"
  Get_PU/1 -> Add4/1
  Data Type Conversion4/1 -> Delay1/1
  Selector/1 -> Get_PU/1
  PhaseCurr/1 -> Data Type Conversion4/1
  Data Type Conversion2/1 -> Delay2/1
  Delay2/1 -> Mod/1
  Constant/1 -> Mod/2
  Mod/1 -> Gain/1
  Data Type Conversion1/1 -> PhaseCurr_fb/1
  Info/1 -> Data Type Conversion2/1
  Mux/1 -> Position_fb/1
  Gain/1 -> Mux/1
  Step/1 -> Data Type Conversion3/1
  Data Type Conversion3/1 -> Mux/2

== system mcb_microchip_pmsm_parameter_est_SAME70/Microcontroller/Application/Param Est/DebugSignals ==
  MotorParams : Inport
  HWInputs : Inport  Port=2
  RsLog : Inport  Port=3
  LdLog : Inport  Port=4
  LqLog : Inport  Port=5
  MechLog : Inport  Port=6
  ActiveTest : Inport  Port=7
  Bus Creator : BusCreator  Inputs=7
  DebugData : Outport
  wires:
  Bus Creator/1 -> DebugData/1
  MotorParams/1 -> Bus Creator/1  "MotorParams"
  MechLog/1 -> Bus Creator/6  "MechLog"
  LqLog/1 -> Bus Creator/5  "LqLog"
  LdLog/1 -> Bus Creator/4  "LdLog"
  RsLog/1 -> Bus Creator/3  "RsLog"
  HWInputs/1 -> Bus Creator/2  "HWInputs"
  ActiveTest/1 -> Bus Creator/7  "ActiveTest"

== system mcb_microchip_pmsm_parameter_est_SAME70/Microcontroller/Application/Param Est/Init ==
  Enable : EnablePort
  Constant : Constant  Value=[0 0 0]  OutDataTypeStr=dataType
  Out1 : Outport  InitialOutput=[0 0 0]
  wires:
  Constant/1 -> Out1/1

== system mcb_microchip_pmsm_parameter_est_SAME70/Microcontroller/Application/Param Est/LdTest ==
  HWInputs : Inport
  MotorParams : Inport  Port=2
  StartEst : Inport  Port=3
  Config : Inport  Port=4
  Enable : EnablePort  StatesWhenEnabling=reset
  Bus Selector : BusSelector  OutputSignals=Iabc
  Bus Selector1 : BusSelector  OutputSignals=Rs
  Ld Estimator : mcbpmsmparamestlib/Ld Estimator
  Vabc : Outport
  Ld : Outport  Port=2
  Log : Outport  Port=3
  wires:
  Config/1 -> Ld Estimator/4
  MotorParams/1 -> Bus Selector1/1
  HWInputs/1 -> Bus Selector/1
  Bus Selector1/1 -> Ld Estimator/2  "<Rs>"
  Bus Selector/1 -> Ld Estimator/1  "<Iabc>"
  Ld Estimator/3 -> Log/1
  Ld Estimator/2 -> Ld/1
  Ld Estimator/1 -> Vabc/1
  StartEst/1 -> Ld Estimator/3

== system mcb_microchip_pmsm_parameter_est_SAME70/Microcontroller/Application/Param Est/LqTest ==
  HWInputs : Inport
  MotorParams : Inport  Port=2
  StartEst : Inport  Port=3
  Config : Inport  Port=4
  Enable : EnablePort  StatesWhenEnabling=reset
  Bus Selector : BusSelector  OutputSignals=Iabc
  Bus Selector1 : BusSelector  OutputSignals=Rs
  Lq Estimator : mcbpmsmparamestlib/Lq Estimator
  Vabc : Outport
  Lq : Outport  Port=2
  Log : Outport  Port=3
  wires:
  Lq Estimator/1 -> Vabc/1
  HWInputs/1 -> Bus Selector/1
  MotorParams/1 -> Bus Selector1/1
  Lq Estimator/2 -> Lq/1
  Lq Estimator/3 -> Log/1
  Config/1 -> Lq Estimator/4
  Bus Selector1/1 -> Lq Estimator/2  "<Rs>"
  Bus Selector/1 -> Lq Estimator/1  "<Iabc>"
  StartEst/1 -> Lq Estimator/3

== system mcb_microchip_pmsm_parameter_est_SAME70/Microcontroller/Application/Param Est/MechParam ==
  HWInputs : Inport
  MotorParams : Inport  Port=2
  StartEst : Inport  Port=3
  Config : Inport  Port=4
  Enable : EnablePort  StatesWhenEnabling=reset
  Bus Selector : BusSelector  OutputSignals=Rs,Ld
  Bus Selector3 : BusSelector  OutputSignals=Iabc,Vdc,Theta,Speed,EnClosedLoop
  Mechanical Parameter Estimator : mcbpmsmparamestlib/Mechanical Parameter Estimator
  Select J : Subsystem  Variant=on  VariantControlMode=sim codegen switching
  Vabc : Outport
  Ke : Outport  Port=2
  J : Outport  Port=3
  B : Outport  Port=4
  InverterEn : Outport  Port=5  OutputWhenDisabled=reset  InitialOutput=1
  Log : Outport  Port=6
  wires:
  Bus Selector/1 -> Mechanical Parameter Estimator/5  "<Rs>"
  MotorParams/1 -> Bus Selector/1
  Config/1 -> Mechanical Parameter Estimator/9
  Bus Selector/2 -> Mechanical Parameter Estimator/6  "<Ld>"
  Mechanical Parameter Estimator/2 -> Ke/1
  Mechanical Parameter Estimator/4 -> B/1
  Mechanical Parameter Estimator/1 -> Vabc/1
  HWInputs/1 -> Bus Selector3/1
  Bus Selector3/1 -> Mechanical Parameter Estimator/1  "<Iabc>"
  Bus Selector3/2 -> Mechanical Parameter Estimator/2  "<Vdc>"
  Mechanical Parameter Estimator/6 -> Log/1
  Mechanical Parameter Estimator/5 -> InverterEn/1
  Bus Selector3/5 -> Mechanical Parameter Estimator/7  "<EnClosedLoop>"
  StartEst/1 -> Mechanical Parameter Estimator/8
  Bus Selector3/3 -> Mechanical Parameter Estimator/3  "<Theta>"
  Bus Selector3/4 -> Mechanical Parameter Estimator/4  "<Speed>"
  Select J/1(Jout) -> J/1
  Mechanical Parameter Estimator/3 -> Select J/1(Jin)

== system mcb_microchip_pmsm_parameter_est_SAME70/Microcontroller/Application/Param Est/RsTest ==
  HWInputs : Inport
  StartEst : Inport  Port=2
  Config : Inport  Port=3
  Enable : EnablePort  StatesWhenEnabling=reset
  Bus Selector : BusSelector  OutputSignals=Iabc,Vdc
  Rs Estimator : mcbpmsmparamestlib/Rs Estimator
  Vabc : Outport
  Rs : Outport  Port=2
  Log : Outport  Port=3
  wires:
  Rs Estimator/1 -> Vabc/1
  HWInputs/1 -> Bus Selector/1
  Rs Estimator/2 -> Rs/1
  Rs Estimator/3 -> Log/1
  Bus Selector/1 -> Rs Estimator/1  "<Iabc>"
  Bus Selector/2 -> Rs Estimator/2  "<Vdc>"
  Config/1 -> Rs Estimator/4
  StartEst/1 -> Rs Estimator/3

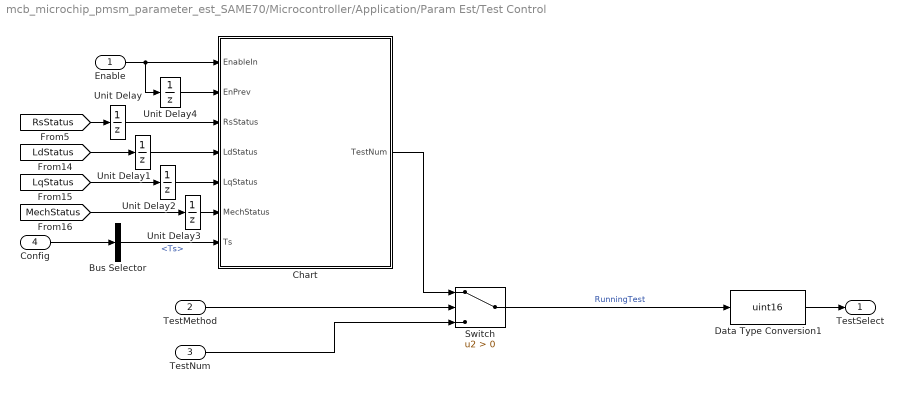
== system mcb_microchip_pmsm_parameter_est_SAME70/Microcontroller/Application/Param Est/Test Control ==
  Enable : Inport
  TestMethod : Inport  Port=2
  TestNum : Inport  Port=3
  Config : Inport  Port=4
  Bus Selector : BusSelector  OutputSignals=Ts
  Chart : Stateflow chart  TreatAsAtomicUnit=on
  Data Type Conversion1 : DataTypeConversion  OutDataTypeStr=uint16  RndMeth=Simplest  SaturateOnIntegerOverflow=off
  Switch : Switch  Criteria=u2 > Threshold  SaturateOnIntegerOverflow=off  InputSameDT=off
  Unit Delay{,1..4} (5 alike) : UnitDelay  SampleTime=-1  HasFrameUpgradeWarning=on
  TestSelect : Outport
  wires:
  Chart/1(TestNum) -> Switch/1
  Enable/1 -> Unit Delay4/1, Chart/1(EnableIn)
  [RsStatus] -> Unit Delay/1
  [LdStatus] -> Unit Delay1/1
  [LqStatus] -> Unit Delay2/1
  [MechStatus] -> Unit Delay3/1
  Unit Delay/1 -> Chart/3(RsStatus)
  Unit Delay1/1 -> Chart/4(LdStatus)
  Unit Delay2/1 -> Chart/5(LqStatus)
  Unit Delay3/1 -> Chart/6(MechStatus)
  Unit Delay4/1 -> Chart/2(EnPrev)
  TestMethod/1 -> Switch/2
  TestNum/1 -> Switch/3
  Switch/1 -> Data Type Conversion1/1  "RunningTest"
  Data Type Conversion1/1 -> TestSelect/1
  Config/1 -> Bus Selector/1
  Bus Selector/1 -> Chart/7(Ts)  "<Ts>"

== system mcb_microchip_pmsm_parameter_est_SAME70/Microcontroller/Application Abstraction/Variant Subsystem/Index Absent ==
  eQEPCnt : Inport
  eQEPIndex : Inport  Port=2
  Mode : Inport  Port=3
  Compare To Constant : simulink/Logic and Bit Operations/Compare To Constant  relop=>=  const=2  OutDataTypeStr=boolean
  Compare To Constant1 : simulink/Logic and Bit Operations/Compare To Constant  relop=<  const=2  OutDataTypeStr=boolean
  Enabled Subsystem : Subsystem  TreatAsAtomicUnit=on
  IIR Filter4 : mcbcontrolslib/IIR Filter  VariantControl=Low Pass Filter  VariantSelect=Low-pass  Filter_constant=0.01  advancedSettings=off  Ts=50e-6  cutOff_freq=32.1525
  Mechanical to Electrical Position : mcbpositiondecoderlib/Mechanical to Electrical Position  PolePairsInputType=Specify via dialog  NrPP=pmsm.p  selectedRange=Radians  MechOfstInputType=Input port  mechOffsetIn=0  maxAngleIn=2*pi  InputDataType=dataType  VariantSelect=floating-point
  Quadrature Decoder : mcbpositiondecoderlib/Quadrature Decoder  EncoderSlitsPerRevolution=pmsm.QEPSlits  EncoderCountsPerSlit=4  CounterSize=16 bits  ExternalIndexCount=off  PositionUnit=Radians  PositionDataType=dataType  ParameterInputType=off  CountsPerRevInverseDataType=single
  Speed Measurement : mcbpositiondecoderlib/Speed Measurement  PositionUnit=Radians  PositionScalingDatatype=uint32  SpeedCalculationMode=Time interval for speed calculation  SampleTimeAsync=Ts  MaximumApplicationSpeed=60000  SpeedResolution=5e-6  DelayLength=20  MaximumMeasurableSpeed=29999  MeasurableSpeedResolution=1.397e-05  SpeedUnit=RPM  PerUnitSpeed=PU_System.N_base  SpeedDataType=dataType
  Terminator : Terminator
  Theta : Outport
  Speed : Outport  Port=2
  EnClosedLoop : Outport  Port=3
  wires:
  eQEPIndex/1 -> Terminator/1
  Compare To Constant/1 -> EnClosedLoop/1
  Mode/1 -> Compare To Constant1/1, Compare To Constant/1
  eQEPCnt/1 -> Quadrature Decoder/1
  Quadrature Decoder/1 -> Speed Measurement/1, Enabled Subsystem/1(In1), Mechanical to Electrical Position/1
  Mechanical to Electrical Position/1 -> Theta/1
  Compare To Constant1/1 -> Enabled Subsystem/Enable
  Enabled Subsystem/1(Out1) -> Mechanical to Electrical Position/2
  Speed Measurement/1 -> IIR Filter4/1
  IIR Filter4/1 -> Speed/1

== system mcb_microchip_pmsm_parameter_est_SAME70/Microcontroller/Application Abstraction/Variant Subsystem/Index Present ==
  eQEPCnt : Inport
  eQEPIndex : Inport  Port=2
  Mode : Inport  Port=3
  Theta : Outport
  Speed : Outport  Port=2
  EnClosedLoop : Outport  Port=3

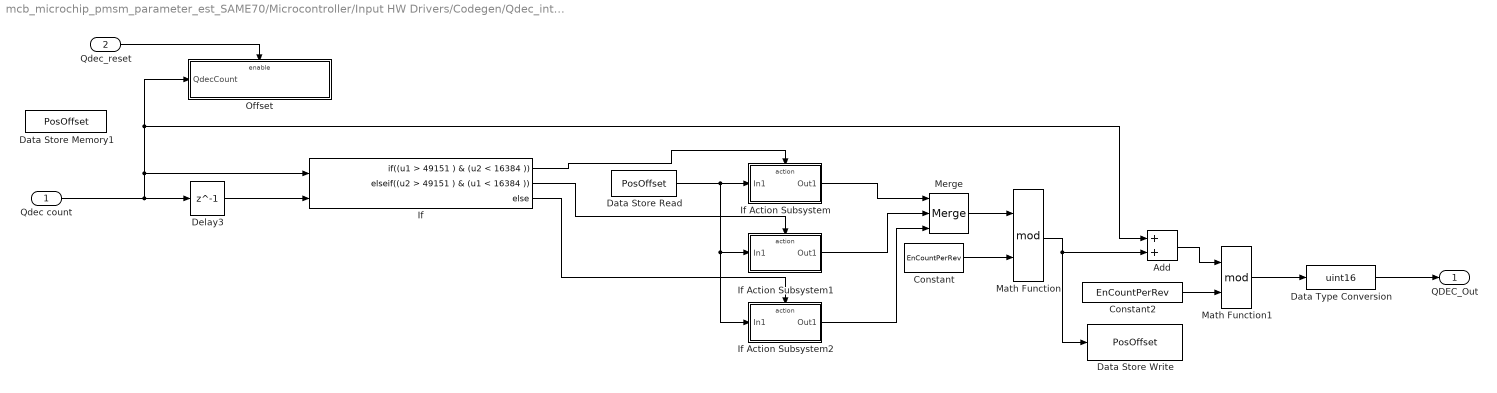
== system mcb_microchip_pmsm_parameter_est_SAME70/Microcontroller/Input HW Drivers/Codegen/Qdec_interface ==
  Qdec count : Inport
  Qdec_reset : Inport  Port=2  OutDataTypeStr=boolean
  Add : Sum  OutDataTypeStr=single
  Constant : Constant  Value=EnCountPerRev  OutDataTypeStr=Inherit: Inherit via back propagation
  Constant2 : Constant  Value=EnCountPerRev  OutDataTypeStr=Inherit: Inherit via back propagation
  Data Store Memory1 : DataStoreMemory  DataStoreName=PosOffset  ShowAdditionalParam=off  OutDataTypeStr=uint16
  Data Store Read : DataStoreRead  DataStoreName=PosOffset  IndexOptions=Index vector (dialog)  Indices=1  OutputSizes=1
  Data Store Write : DataStoreWrite  DataStoreName=PosOffset  IndexOptions=Index vector (dialog)  Indices=1  OutputSizes=1
  Data Type Conversion : DataTypeConversion  OutDataTypeStr=uint16  SaturateOnIntegerOverflow=off  RndMeth=Floor
  Delay3 : Delay  DelayLength=1  InitialCondition=0
  If : If  NumInputs=2  IfExpression=(u1 > 49151 ) & (u2 < 16384 )  ElseIfExpressions=(u2 > 49151 ) & (u1 < 16384 )
  If Action Subsystem : Subsystem  TreatAsAtomicUnit=on
  If Action Subsystem1 : Subsystem  TreatAsAtomicUnit=on
  If Action Subsystem2 : Subsystem  TreatAsAtomicUnit=on
  Math Function : Math  Operator=mod  SignedPower=on
  Math Function1 : Math  Operator=mod  SignedPower=on
  Merge : Merge  Inputs=3
  Offset : Subsystem
  QDEC_Out : Outport
  wires:
  Qdec count/1 -> Offset/1(QdecCount), Add/1, If/1, Delay3/1
  If Action Subsystem2/1(Out1) -> Merge/3
  If/2 -> If Action Subsystem1/Action
  If Action Subsystem1/1(Out1) -> Merge/2
  Data Store Read/1 -> If Action Subsystem2/1(In1), If Action Subsystem1/1(In1), If Action Subsystem/1(In1)
  If/3 -> If Action Subsystem2/Action
  If Action Subsystem/1(Out1) -> Merge/1
  Constant/1 -> Math Function/2
  Delay3/1 -> If/2
  Merge/1 -> Math Function/1
  If/1 -> If Action Subsystem/Action
  Math Function/1 -> Data Store Write/1, Add/2
  Add/1 -> Math Function1/1
  Constant2/1 -> Math Function1/2
  Math Function1/1 -> Data Type Conversion/1
  Qdec_reset/1 -> Offset/Enable
  Data Type Conversion/1 -> QDEC_Out/1

== system mcb_microchip_pmsm_parameter_est_SAME70/Microcontroller/Input Scaling/Variant Subsystem/Automatic offset calibration ==
  Mode : Inport
  Iab_ADC : Inport  Port=2
  Add : Sum  Inputs=-+  RndMeth=Simplest  OutDataTypeStr=Inherit: Same as first input
  Compare To Constant : simulink/Logic and Bit Operations/Compare To Constant  relop=<  const=1  OutDataTypeStr=boolean
  Data Type Conversion : DataTypeConversion  OutDataTypeStr=int32  ConvertRealWorld=Stored Integer (SI)  RndMeth=Simplest  SaturateOnIntegerOverflow=off
  Enabled Subsystem : Subsystem  TreatAsAtomicUnit=on
  Gain : Gain  Gain=inverter.AmpPerCount  OutDataTypeStr=dataType  RndMeth=Simplest
  Iab : Outport
  wires:
  Data Type Conversion/1 -> Add/2, Enabled Subsystem/1(In1)
  Gain/1 -> Iab/1
  Enabled Subsystem/1(Out1) -> Add/1
  Add/1 -> Gain/1
  Compare To Constant/1 -> Enabled Subsystem/Enable
  Mode/1 -> Compare To Constant/1
  Iab_ADC/1 -> Data Type Conversion/1

== system mcb_microchip_pmsm_parameter_est_SAME70/Microcontroller/Input Scaling/Variant Subsystem/Offser via parameter ==
  Mode : Inport
  Iab_ADC : Inport  Port=2
  Add : Sum  Inputs=-+  RndMeth=Simplest  OutDataTypeStr=Inherit: Same as first input
  Constant : Constant  Value=[inverter.CtSensAOffset inverter.CtSensBOffset]  OutDataTypeStr=Inherit: Inherit via back propagation
  Gain : Gain  Gain=inverter.AmpPerCount  OutDataTypeStr=dataType  RndMeth=Simplest
  Terminator : Terminator
  Iab : Outport
  wires:
  Gain/1 -> Iab/1
  Iab_ADC/1 -> Add/2
  Add/1 -> Gain/1
  Constant/1 -> Add/1
  Mode/1 -> Terminator/1

== system mcb_microchip_pmsm_parameter_est_SAME70/Microcontroller/Output PWM Drivers/Sim/Subsystem ==
  PWM_In : Inport
  Constant : Constant  Value=0.5  OutDataTypeStr=dataType
  Gain : Gain  Gain=0.5  OutDataTypeStr=Inherit: Same as input
  Sum : Sum  Inputs=|++
  PWM_Duty_Cycles : Outport
  wires:
  Gain/1 -> Sum/1
  Constant/1 -> Sum/2
  PWM_In/1 -> Gain/1
  Sum/1 -> PWM_Duty_Cycles/1  "PWM_Duty_Cycles"

== system mcb_microchip_pmsm_parameter_est_SAME70/Microcontroller/SCI In Abstraction/Variant Subsystem/Codegen ==
  SCI_Data : Inport
  Mode : Inport  Port=2
  AND : Logic  IconShape=distinctive  AllPortsSameDT=off  OutDataTypeStr=boolean
  Bus Creator : BusCreator  Inputs=4
  Byte Unpack1 : svdutilitieslib/Byte Unpack  dimensions={[1]}  datatypes={'single'}  byteAlign=1  blockPlatform=tic2000
      settings: LibrarySourceBlock=c2000lib/Target Communication/Byte Unpack
  Compare To Constant : simulink/Logic and Bit Operations/Compare To Constant  relop=>=  const=2  OutDataTypeStr=boolean
  Demux : Demux  Outputs=8
  Mux : Mux
  Subsystem1 : Subsystem
  Terminator : Terminator
  Terminator1 : Terminator
  Terminator2 : Terminator
  ConfigAndCommand : Outport
  DebugSel : Outport  Port=2
  wires:
  Bus Creator/1 -> ConfigAndCommand/1
  AND/1 -> Bus Creator/1  "Enable"
  Subsystem1/1(Enable) -> AND/2
  Compare To Constant/1 -> AND/1
  Mode/1 -> Compare To Constant/1
  SCI_Data/1 -> Demux/1
  Demux/1 -> Subsystem1/1(Count)
  Subsystem1/5(DebugSelect) -> DebugSel/1
  Subsystem1/2(TestMethod) -> Bus Creator/2  "TestMethod"
  Subsystem1/3(TestSelect) -> Bus Creator/3  "TestSelect"
  Subsystem1/4(Config) -> Bus Creator/4  "Config"
  Mux/1 -> Byte Unpack1/1
  Demux/5 -> Mux/4
  Demux/3 -> Mux/2
  Demux/2 -> Mux/1
  Demux/4 -> Mux/3
  Byte Unpack1/1 -> Subsystem1/2(Data)
  Demux/6 -> Terminator/1
  Demux/8 -> Terminator1/1
  Demux/7 -> Terminator2/1

== system mcb_microchip_pmsm_parameter_est_SAME70/Microcontroller/SCI In Abstraction/Variant Subsystem/Sim ==
  SCI_Data : Inport
  Mode : Inport  Port=2
  AND : Logic  IconShape=distinctive  AllPortsSameDT=off  OutDataTypeStr=boolean
  Bus Creator : BusCreator  Inputs=4
  Compare To Constant : simulink/Logic and Bit Operations/Compare To Constant  relop=>=  const=2  OutDataTypeStr=boolean
  DebugDataSelect : Constant  OutDataTypeStr=uint16
  Parameter Estimation Configurator : mcbpmsmparamestlib/Parameter Estimation Configurator  P=pmsm.p  NRated=pmsm.N_rated  IRated=pmsm.I_rated  ImaxInverter=inverter.ISenseMax  RBoard=inverter.R_board  ISenseGain=inverter.AmpPerCount  VSenseGain=inverter.VoltPerCount  FreqMax=1000  FreqMin=200  FreqStepSweep=100  FreqStepEst=10  FreqNum=10  KeTime=5  KeSpeed=pmsm.N_rated * 0.9  IqRefFOC=0.2  KpKiInputEnable=off  Kp=1  Ki=10  JSpeedLow=pmsm.N_rated * 0.2  DataType=single  Ts=Ts
  Terminator : Terminator
  Test Enable : Step  Time=3  OutDataTypeStr=single
  Test Method : Constant  OutDataTypeStr=Inherit: Inherit via back propagation
  Test Select : Constant  Value=0  OutDataTypeStr=uint16
  ConfigAndCommand : Outport
  DebugSel : Outport  Port=2
  wires:
  SCI_Data/1 -> Terminator/1
  Mode/1 -> Compare To Constant/1
  Compare To Constant/1 -> AND/1
  Test Enable/1 -> AND/2
  Bus Creator/1 -> ConfigAndCommand/1
  AND/1 -> Bus Creator/1  "Enable"
  DebugDataSelect/1 -> DebugSel/1
  Test Method/1 -> Bus Creator/2  "TestMethod"
  Test Select/1 -> Bus Creator/3  "TestSelect"
  Parameter Estimation Configurator/1 -> Bus Creator/4  "Config"

== system mcb_microchip_pmsm_parameter_est_SAME70/Microcontroller/SCI_Rx/CodeGen/Subsystem ==
  In1 : Inport
  Enable1 : EnablePort
  Data : Outport
  wires:
  In1/1 -> Data/1
